simulink model "parkingNavigationTest"  (R2021b)
settings: Solver=VariableStepAuto  StartTime=0.0  StopTime=3600  FixedStep=0.01  RelTol=1e-3
model workspace (MAT data in the model file):
  enableTransmit = 1
libraries: matrix_library x10, sharedutil x4, simulink x3, aerolibutil x2
(part 1 of 2)
settings Model: Creator=Vladik  LastModifiedBy=Vladik

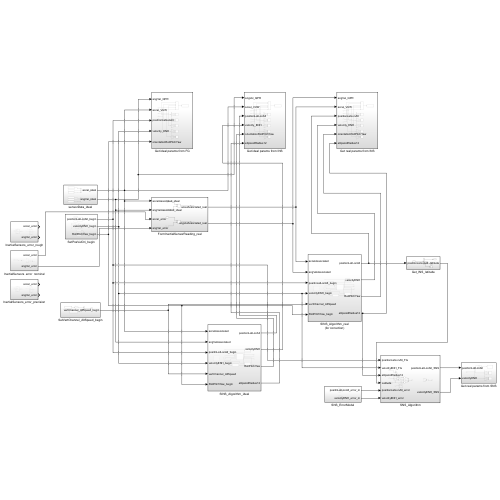
[thumbnail: Simulink's stored preview of the top-level diagram]
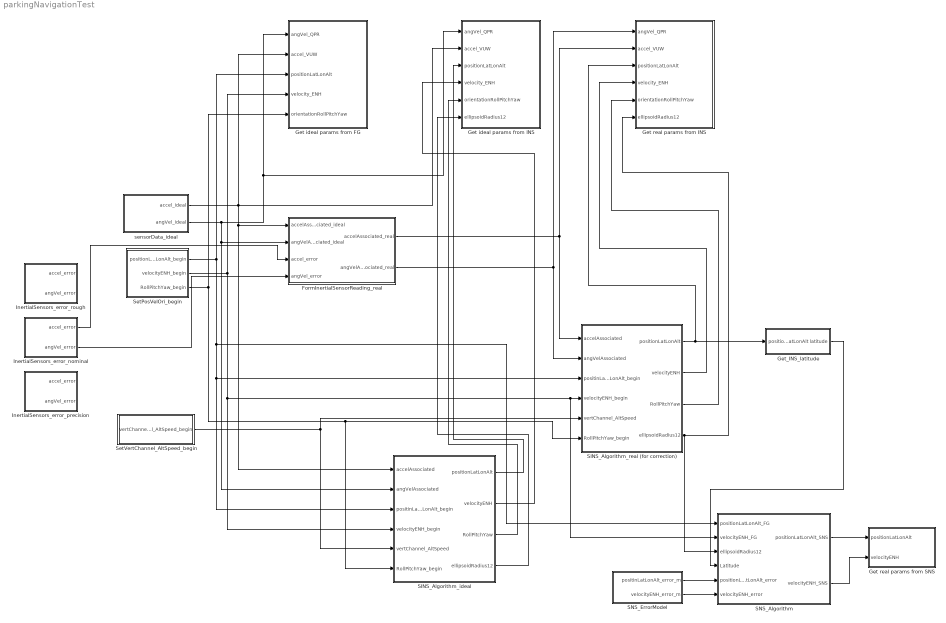
== system parkingNavigationTest ==
  FormInertialSensorReading_real : Subsystem
  Get ideal params from FG : Subsystem
  Get ideal params from INS : Subsystem
  Get real params from INS : Subsystem
  Get real params from SNS : Subsystem
  Get_INS_latitude : Subsystem
  InertialSensors_error_nominal : Subsystem
  InertialSensors_error_precision : Subsystem
  InertialSensors_error_rough : Subsystem
  SINS_Algorithm_ideal : Subsystem
  SINS_Algorithm_real (for correction) : Subsystem
  SNS_Algorithm : Subsystem
  SNS_ErrorModel : Subsystem
  SetPosVelOri_begin : Subsystem
  SetVertChannel_AltSpeed_begin : Subsystem
  sensorData_ideal : Subsystem
  wires:
  SetPosVelOri_begin/2(velocityENH_begin) -> SNS_Algorithm/2(velocityENH_FG), SINS_Algorithm_real (for correction)/4(velocityENH_begin), SINS_Algorithm_ideal/4(velocityENH_begin), Get ideal params from FG/4(velocity_ENH)
  InertialSensors_error_nominal/1(accel_error) -> FormInertialSensorReading_real/3(accel_error)
  InertialSensors_error_nominal/2(angVel_error) -> FormInertialSensorReading_real/4(angVel_error)
  FormInertialSensorReading_real/1(accelAssociated_real) -> SINS_Algorithm_real (for correction)/1(accelAssociated), Get real params from INS/2(accel_VUW)
  FormInertialSensorReading_real/2(angVelAssociated_real) -> SINS_Algorithm_real (for correction)/2(angVelAssociated), Get real params from INS/1(angVel_QPR)
  SetPosVelOri_begin/3(RollPitchYaw_begin) -> SINS_Algorithm_ideal/6(RollPitchYaw_begin), SINS_Algorithm_real (for correction)/6(RollPitchYaw_begin), Get ideal params from FG/5(orientationRollPitchYaw)
  SetPosVelOri_begin/1(positionLatLonAlt_begin) -> SINS_Algorithm_ideal/3(positinLatLonAlt_begin), SINS_Algorithm_real (for correction)/3(positinLatLonAlt_begin), SNS_Algorithm/1(positionLatLonAlt_FG), Get ideal params from FG/3(positionLatLonAlt)
  sensorData_ideal/1(accel_ideal) -> SINS_Algorithm_ideal/1(accelAssociated), FormInertialSensorReading_real/1(accelAssociated_ideal), Get ideal params from FG/2(accel_VUW), Get ideal params from INS/2(accel_VUW)
  SINS_Algorithm_ideal/1(positionLatLonAlt) -> Get ideal params from INS/3(positionLatLonAlt)
  SINS_Algorithm_ideal/2(velocityENH) -> Get ideal params from INS/4(velocity_ENH)
  SINS_Algorithm_ideal/3(RollPitchYaw) -> Get ideal params from INS/5(orientationRollPitchYaw)
  SINS_Algorithm_real (for correction)/1(positionLatLonAlt) -> Get_INS_latitude/1(positionLatLonAlt), Get real params from INS/3(positionLatLonAlt)
  SINS_Algorithm_real (for correction)/3(RollPitchYaw) -> Get real params from INS/5(orientationRollPitchYaw)
  SetVertChannel_AltSpeed_begin/1(vertChannel_AltSpeed_begin) -> SINS_Algorithm_ideal/5(vertChannel_AltSpeed), SINS_Algorithm_real (for correction)/5(vertChannel_AltSpeed)
  SINS_Algorithm_real (for correction)/2(velocityENH) -> Get real params from INS/4(velocity_ENH)
  sensorData_ideal/2(angVel_ideal) -> SINS_Algorithm_ideal/2(angVelAssociated), FormInertialSensorReading_real/2(angVelAssociated_ideal), Get ideal params from INS/1(angVel_QPR), Get ideal params from FG/1(angVel_QPR)
  SINS_Algorithm_ideal/4(ellipsoidRadius12) -> Get ideal params from INS/6(ellipsoidRadius12)
  SINS_Algorithm_real (for correction)/4(ellipsoidRadius12) -> SNS_Algorithm/3(ellipsoidRadius12), Get real params from INS/6(ellipsoidRadius12)
  SNS_ErrorModel/1(positinLatLonAlt_error_m) -> SNS_Algorithm/5(positionLatLonAlt_error)
  SNS_ErrorModel/2(velocityENH_error_m) -> SNS_Algorithm/6(velocityENH_error)
  Get_INS_latitude/1(latitude) -> SNS_Algorithm/4(Latitude)
  SNS_Algorithm/1(positionLatLonAlt_SNS) -> Get real params from SNS/1(positionLatLonAlt)
  SNS_Algorithm/2(velocityENH_SNS) -> Get real params from SNS/2(velocityENH)

== system parkingNavigationTest/FormInertialSensorReading_real ==
  accelAssociated_ideal : Inport
  angVelAssociated_ideal : Inport  Port=2
  accel_error : Inport  Port=3
  angVel_error : Inport  Port=4
  Add : Sum
  Add1 : Sum
  accelAssociated_real : Outport
  angVelAssociated_real : Outport  Port=2
  wires:
  accelAssociated_ideal/1 -> Add/1
  accel_error/1 -> Add/2
  Add/1 -> accelAssociated_real/1
  Add1/1 -> angVelAssociated_real/1
  angVelAssociated_ideal/1 -> Add1/1
  angVel_error/1 -> Add1/2

== system parkingNavigationTest/Get ideal params from FG ==
  angVel_QPR : Inport
  accel_VUW : Inport  Port=2
  positionLatLonAlt : Inport  Port=3
  velocity_ENH : Inport  Port=4
  orientationRollPitchYaw : Inport  Port=5
  Demux{1..5} (5 alike) : Demux  Outputs=3
  Vector Concatenate2 : Concatenate  NumInputs=5  Mode=Multidimensional array
  Write Ideal To File : ToFile  Filename=x_ideal_fg.mat  MatrixName=x_ideal_fg
  dispAccelerationIdeal : Scope  NumInputPorts=3
  dispAngularVelocityIdeal : Scope  NumInputPorts=3
  dispOrientationIdeal : Scope  NumInputPorts=3
  dispPositionIdeal : Scope  NumInputPorts=3
  dispVelocityIdeal : Scope  NumInputPorts=3
  wires:
  Demux3/1 -> dispPositionIdeal/1
  Demux3/3 -> dispPositionIdeal/3
  Demux3/2 -> dispPositionIdeal/2
  positionLatLonAlt/1 -> Demux3/1, Vector Concatenate2/3
  Demux4/1 -> dispVelocityIdeal/1
  Demux4/3 -> dispVelocityIdeal/3
  Demux4/2 -> dispVelocityIdeal/2
  velocity_ENH/1 -> Vector Concatenate2/4, Demux4/1
  Demux5/1 -> dispOrientationIdeal/1
  Demux5/2 -> dispOrientationIdeal/2
  Demux5/3 -> dispOrientationIdeal/3
  orientationRollPitchYaw/1 -> Vector Concatenate2/5, Demux5/1
  Demux1/3 -> dispAccelerationIdeal/3
  Demux1/1 -> dispAccelerationIdeal/1
  Demux1/2 -> dispAccelerationIdeal/2
  accel_VUW/1 -> Demux1/1, Vector Concatenate2/2
  Demux2/3 -> dispAngularVelocityIdeal/3
  Demux2/1 -> dispAngularVelocityIdeal/1
  Demux2/2 -> dispAngularVelocityIdeal/2
  angVel_QPR/1 -> Vector Concatenate2/1, Demux2/1
  Vector Concatenate2/1 -> Write Ideal To File/1

== system parkingNavigationTest/Get ideal params from INS ==
  angVel_QPR : Inport
  accel_VUW : Inport  Port=2
  positionLatLonAlt : Inport  Port=3
  velocity_ENH : Inport  Port=4
  orientationRollPitchYaw : Inport  Port=5
  ellipsoidRadius12 : Inport  Port=6
  Demux{1..5} (5 alike) : Demux  Outputs=3
  Vector Concatenate2 : Concatenate  NumInputs=6  Mode=Multidimensional array
  Write Ideal To File : ToFile  Filename=x_ideal_ins.mat  MatrixName=x_ideal_ins
  dispAccelerationIdeal_INS : Scope  NumInputPorts=3
  dispAngularVelocityIdeal_INS : Scope  NumInputPorts=3
  dispOrientationIdeal_INS : Scope  NumInputPorts=3
  dispPositionIdeal_INS : Scope  NumInputPorts=3
  dispVelocityIdeal_INS : Scope  NumInputPorts=3
  wires:
  Demux3/1 -> dispPositionIdeal_INS/1
  Demux3/3 -> dispPositionIdeal_INS/3
  Demux3/2 -> dispPositionIdeal_INS/2
  positionLatLonAlt/1 -> Vector Concatenate2/3, Demux3/1
  Demux4/1 -> dispVelocityIdeal_INS/1
  Demux4/3 -> dispVelocityIdeal_INS/3
  Demux4/2 -> dispVelocityIdeal_INS/2
  velocity_ENH/1 -> Vector Concatenate2/4, Demux4/1
  Demux5/1 -> dispOrientationIdeal_INS/1
  Demux5/2 -> dispOrientationIdeal_INS/2
  Demux5/3 -> dispOrientationIdeal_INS/3
  orientationRollPitchYaw/1 -> Vector Concatenate2/5, Demux5/1
  Demux1/3 -> dispAccelerationIdeal_INS/3
  Demux1/1 -> dispAccelerationIdeal_INS/1
  Demux1/2 -> dispAccelerationIdeal_INS/2
  accel_VUW/1 -> Vector Concatenate2/2, Demux1/1
  Demux2/3 -> dispAngularVelocityIdeal_INS/3
  Demux2/1 -> dispAngularVelocityIdeal_INS/1
  Demux2/2 -> dispAngularVelocityIdeal_INS/2
  angVel_QPR/1 -> Vector Concatenate2/1, Demux2/1
  Vector Concatenate2/1 -> Write Ideal To File/1
  ellipsoidRadius12/1 -> Vector Concatenate2/6

== system parkingNavigationTest/Get real params from INS ==
  angVel_QPR : Inport
  accel_VUW : Inport  Port=2
  positionLatLonAlt : Inport  Port=3
  velocity_ENH : Inport  Port=4
  orientationRollPitchYaw : Inport  Port=5
  ellipsoidRadius12 : Inport  Port=6
  Demux{1..5} (5 alike) : Demux  Outputs=3
  Vector Concatenate2 : Concatenate  NumInputs=6  Mode=Multidimensional array
  Write Real To File : ToFile  Filename=x_real_ins.mat  MatrixName=x_real_ins
  dispAccelerationReal_INS : Scope  NumInputPorts=3
  dispAngularVelocityReal_INS : Scope  NumInputPorts=3
  dispOrientationReal_INS : Scope  NumInputPorts=3
  dispPositionReal_INS : Scope  NumInputPorts=3
  dispVelocityReal_INS : Scope  NumInputPorts=3
  wires:
  Demux3/1 -> dispPositionReal_INS/1
  Demux3/3 -> dispPositionReal_INS/3
  Demux3/2 -> dispPositionReal_INS/2
  positionLatLonAlt/1 -> Vector Concatenate2/3, Demux3/1
  Demux4/1 -> dispVelocityReal_INS/1
  Demux4/3 -> dispVelocityReal_INS/3
  Demux4/2 -> dispVelocityReal_INS/2
  velocity_ENH/1 -> Vector Concatenate2/4, Demux4/1
  Demux5/1 -> dispOrientationReal_INS/1
  Demux5/2 -> dispOrientationReal_INS/2
  Demux5/3 -> dispOrientationReal_INS/3
  orientationRollPitchYaw/1 -> Vector Concatenate2/5, Demux5/1
  Demux1/3 -> dispAccelerationReal_INS/3
  Demux1/1 -> dispAccelerationReal_INS/1
  Demux1/2 -> dispAccelerationReal_INS/2
  accel_VUW/1 -> Vector Concatenate2/2, Demux1/1
  Demux2/3 -> dispAngularVelocityReal_INS/3
  Demux2/1 -> dispAngularVelocityReal_INS/1
  Demux2/2 -> dispAngularVelocityReal_INS/2
  angVel_QPR/1 -> Vector Concatenate2/1, Demux2/1
  Vector Concatenate2/1 -> Write Real To File/1
  ellipsoidRadius12/1 -> Vector Concatenate2/6

== system parkingNavigationTest/Get real params from SNS ==
  positionLatLonAlt : Inport
  velocityENH : Inport  Port=2
  Demux3 : Demux  Outputs=3
  Demux4 : Demux  Outputs=3
  Vector Concatenate2 : Concatenate  Mode=Multidimensional array
  Write Data To File : ToFile  Filename=x_real_sns.mat  MatrixName=x_real_sns
  dispPosition : Scope  NumInputPorts=3
  dispVelocity : Scope  NumInputPorts=3
  wires:
  positionLatLonAlt/1 -> Vector Concatenate2/1, Demux3/1
  Vector Concatenate2/1 -> Write Data To File/1
  Demux3/2 -> dispPosition/2
  Demux3/3 -> dispPosition/3
  Demux3/1 -> dispPosition/1
  velocityENH/1 -> Vector Concatenate2/2, Demux4/1
  Demux4/1 -> dispVelocity/1
  Demux4/2 -> dispVelocity/2
  Demux4/3 -> dispVelocity/3

== system parkingNavigationTest/Get_INS_latitude ==
  positionLatLonAlt : Inport
  Demux : Demux  Outputs=3
  Terminator : Terminator
  Terminator1 : Terminator
  latitude : Outport
  wires:
  positionLatLonAlt/1 -> Demux/1
  Demux/1 -> latitude/1
  Demux/2 -> Terminator/1
  Demux/3 -> Terminator1/1

== system parkingNavigationTest/InertialSensors_error_nominal ==
  Add1 : Sum
  Add4 : Sum
  Mux : Mux  Inputs=3
  Mux1 : Mux  Inputs=3
  Ramp : simulink/Sources/Ramp  slope=0.015*pi/180/3600  start=0  InitialOutput=0
  accelNoise : RandomNumber  Variance=1e-8  SampleTime=1
  accelZeroOffset : Constant  Value=5e-4
  gyroNoise : RandomNumber  Variance=(0.01*pi/180/3600)^2  SampleTime=1
  accel_error : Outport
  angVel_error : Outport  Port=2
  wires:
  gyroNoise/1 -> Add4/2
  accelZeroOffset/1 -> Add1/1
  accelNoise/1 -> Add1/2
  Add1/1 -> Mux/1, Mux/2, Mux/3
  Mux/1 -> accel_error/1
  Mux1/1 -> angVel_error/1
  Ramp/1 -> Add4/1
  Add4/1 -> Mux1/1, Mux1/2, Mux1/3

== system parkingNavigationTest/InertialSensors_error_precision ==
  Add{,1..5} (6 alike) : Sum
  Mux : Mux  Inputs=3
  Mux1 : Mux  Inputs=3
  Ramp : simulink/Sources/Ramp  slope=0.0015*pi/180/3600  start=0  InitialOutput=0
  accelNoise : RandomNumber  Variance=1e-10  SampleTime=1
  accelZeroOffset : Constant  Value=0.00005
  gyroNoise : RandomNumber  Variance=(0.001*pi/180/3600)^2  SampleTime=1
  accel_error : Outport
  angVel_error : Outport  Port=2
  wires:
  gyroNoise/1 -> Add/2, Add5/2, Add4/2
  accelZeroOffset/1 -> Add2/1, Add3/1, Add1/1
  accelNoise/1 -> Add3/2, Add2/2, Add1/2
  Add1/1 -> Mux/2
  Mux/1 -> accel_error/1
  Mux1/1 -> angVel_error/1
  Add2/1 -> Mux/1
  Add3/1 -> Mux/3
  Ramp/1 -> Add5/1, Add4/1, Add/1
  Add4/1 -> Mux1/2
  Add/1 -> Mux1/1
  Add5/1 -> Mux1/3

== system parkingNavigationTest/InertialSensors_error_rough ==
  Add{,1..5} (6 alike) : Sum
  Mux : Mux  Inputs=3
  Mux1 : Mux  Inputs=3
  Ramp : simulink/Sources/Ramp  slope=0.15*pi/180/3600  start=0  InitialOutput=0
  accelNoise : RandomNumber  Variance=1e-6  SampleTime=1
  accelZeroOffset : Constant  Value=5e-3
  gyroNoise : RandomNumber  Variance=(0.1*pi/180/3600)^2  SampleTime=1
  accel_error : Outport
  angVel_error : Outport  Port=2
  wires:
  gyroNoise/1 -> Add/2, Add5/2, Add4/2
  accelZeroOffset/1 -> Add2/1, Add3/1, Add1/1
  accelNoise/1 -> Add3/2, Add2/2, Add1/2
  Add1/1 -> Mux/2
  Mux/1 -> accel_error/1
  Mux1/1 -> angVel_error/1
  Add2/1 -> Mux/1
  Add3/1 -> Mux/3
  Ramp/1 -> Add5/1, Add4/1, Add/1
  Add4/1 -> Mux1/2
  Add/1 -> Mux1/1
  Add5/1 -> Mux1/3

== system parkingNavigationTest/SINS_Algorithm_ideal ==
  accelAssociated : Inport
  angVelAssociated : Inport  Port=2
  positinLatLonAlt_begin : Inport  Port=3
  velocityENH_begin : Inport  Port=4
  vertChannel_AltSpeed : Inport  Port=5
  RollPitchYaw_begin : Inport  Port=6
  CalculateAccelerationsXYZ : Subsystem
  GetC_begin_easy : Subsystem
  GetC_begin_vectorMatching : Subsystem  Commented=on
  NavigationAlgorithm : Subsystem
  OrientationAlgorithm : Subsystem
  U_earth : Constant  Value=7.29212e-5
  removeVelocityH : Subsystem
  positionLatLonAlt : Outport
  velocityENH : Outport  Port=2
  RollPitchYaw : Outport  Port=3
  ellipsoidRadius12 : Outport  Port=4
  wires:
  GetC_begin_easy/1(C_assoc_norm_begin) -> OrientationAlgorithm/3(C_assoc_norm_begin)
  velocityENH_begin/1 -> removeVelocityH/1(velocityENH_begin)
  NavigationAlgorithm/4(ellipsoidRadius12) -> ellipsoidRadius12/1
  vertChannel_AltSpeed/1 -> NavigationAlgorithm/5(vertChannel_AltSpeed)
  NavigationAlgorithm/2(velocityENH) -> velocityENH/1
  removeVelocityH/1(velocityEN_begin) -> NavigationAlgorithm/3(velocityEN_begin)
  positinLatLonAlt_begin/1 -> NavigationAlgorithm/2(positionLatLonAlt_begin)
  NavigationAlgorithm/3(angVelNorm_matrix_3x3) -> OrientationAlgorithm/2(angVelNorm_matrix)
  NavigationAlgorithm/1(positionLatLonAlt) -> positionLatLonAlt/1
  U_earth/1 -> NavigationAlgorithm/4(U_earth)
  angVelAssociated/1 -> OrientationAlgorithm/1(angVel_inertial_assoc)
  OrientationAlgorithm/1(C_assoc_norm) -> CalculateAccelerationsXYZ/2(C_accoc_norm)
  accelAssociated/1 -> CalculateAccelerationsXYZ/1(accelerationAssociated)
  RollPitchYaw_begin/1 -> GetC_begin_easy/1(RollPitchYaw_begin)
  OrientationAlgorithm/2(RollPitchYaw) -> RollPitchYaw/1
  CalculateAccelerationsXYZ/1(accelerationXYZ) -> NavigationAlgorithm/1(accelerationXYZ)

== system parkingNavigationTest/SINS_Algorithm_real (for correction) ==
  accelAssociated : Inport
  angVelAssociated : Inport  Port=2
  positinLatLonAlt_begin : Inport  Port=3
  velocityENH_begin : Inport  Port=4
  vertChannel_AltSpeed : Inport  Port=5
  RollPitchYaw_begin : Inport  Port=6
  CalculateAccelerationsXYZ : Subsystem
  GetC_begin_easy : Subsystem
  GetC_begin_vectorMatching : Subsystem  Commented=on
  NavigationAlgorithm : Subsystem
  OrientationAlgorithm : Subsystem
  U_earth : Constant  Value=7.29212e-5
  removeVelocityH : Subsystem
  positionLatLonAlt : Outport
  velocityENH : Outport  Port=2
  RollPitchYaw : Outport  Port=3
  ellipsoidRadius12 : Outport  Port=4
  wires:
  NavigationAlgorithm/2(velocityENH) -> velocityENH/1
  CalculateAccelerationsXYZ/1(accelerationXYZ) -> NavigationAlgorithm/1(accelerationXYZ)
  positinLatLonAlt_begin/1 -> NavigationAlgorithm/2(positionLatLonAlt_begin)
  removeVelocityH/1(velocityEN_begin) -> NavigationAlgorithm/3(velocityEN_begin)
  velocityENH_begin/1 -> removeVelocityH/1(velocityENH_begin)
  GetC_begin_easy/1(C_assoc_norm_begin) -> OrientationAlgorithm/3(C_assoc_norm_begin)
  vertChannel_AltSpeed/1 -> NavigationAlgorithm/5(vertChannel_AltSpeed)
  U_earth/1 -> NavigationAlgorithm/4(U_earth)
  NavigationAlgorithm/4(ellipsoidRadius12) -> ellipsoidRadius12/1
  OrientationAlgorithm/1(C_assoc_norm) -> CalculateAccelerationsXYZ/2(C_accoc_norm)
  accelAssociated/1 -> CalculateAccelerationsXYZ/1(accelerationAssociated)
  NavigationAlgorithm/3(angVelNorm_matrix_3x3) -> OrientationAlgorithm/2(angVelNorm_matrix)
  OrientationAlgorithm/2(RollPitchYaw) -> RollPitchYaw/1
  NavigationAlgorithm/1(positionLatLonAlt) -> positionLatLonAlt/1
  angVelAssociated/1 -> OrientationAlgorithm/1(angVel_inertial_assoc)
  RollPitchYaw_begin/1 -> GetC_begin_easy/1(RollPitchYaw_begin)

== system parkingNavigationTest/SNS_Algorithm ==
  positionLatLonAlt_FG : Inport
  velocityENH_FG : Inport  Port=2
  ellipsoidRadius12 : Inport  Port=3
  Latitude : Inport  Port=4
  positionLatLonAlt_error : Inport  Port=5
  velocityENH_error : Inport  Port=6
  Add1 : Sum
  AltReal_m : Sum
  Cos : Trigonometry  Operator=cos
  Demux1 : Demux  Outputs=3
  Demux7 : Demux  Outputs=3
  Demux8 : Demux  Outputs=2
  Divide : Product  Inputs=*/
  Divide1 : Product  Inputs=*//
  LatSNS_rad : Sum
  LonReal_rad : Sum
  Mux2 : Mux  Inputs=3
  positionLatLonAlt_SNS : Outport
  velocityENH_SNS : Outport  Port=2
  wires:
  Divide1/1 -> LonReal_rad/1
  Divide/1 -> LatSNS_rad/1
  ellipsoidRadius12/1 -> Demux8/1
  positionLatLonAlt_error/1 -> Demux7/1
  Demux7/1 -> Divide/1
  Demux7/2 -> Divide1/1
  Latitude/1 -> Cos/1
  Cos/1 -> Divide1/3
  positionLatLonAlt_FG/1 -> Demux1/1
  Demux1/1 -> LatSNS_rad/2
  Demux1/2 -> LonReal_rad/2
  Demux7/3 -> AltReal_m/1
  Demux1/3 -> AltReal_m/2
  LonReal_rad/1 -> Mux2/2
  LatSNS_rad/1 -> Mux2/1
  AltReal_m/1 -> Mux2/3
  Mux2/1 -> positionLatLonAlt_SNS/1
  velocityENH_FG/1 -> Add1/1
  velocityENH_error/1 -> Add1/2
  Add1/1 -> velocityENH_SNS/1
  Demux8/2 -> Divide/2
  Demux8/1 -> Divide1/2

== system parkingNavigationTest/SNS_ErrorModel ==
  AltError_m : RandomNumber  Variance=100  SampleTime=0.1
  LatError_m : RandomNumber  Variance=100  SampleTime=0.1
  LonError_m : RandomNumber  Variance=100  SampleTime=0.1
  Mux : Mux  Inputs=3
  Mux1 : Mux  Inputs=3
  VelE_error_m : RandomNumber  Variance=0.01  SampleTime=0.1
  VelH_error_m : RandomNumber  Variance=0.01  SampleTime=0.1
  VelN_error_m : RandomNumber  Variance=0.01  SampleTime=0.1
  positinLatLonAlt_error_m : Outport
  velocityENH_error_m : Outport  Port=2
  wires:
  LonError_m/1 -> Mux/2
  LatError_m/1 -> Mux/1
  AltError_m/1 -> Mux/3
  Mux/1 -> positinLatLonAlt_error_m/1
  VelN_error_m/1 -> Mux1/2
  VelE_error_m/1 -> Mux1/1
  VelH_error_m/1 -> Mux1/3
  Mux1/1 -> velocityENH_error_m/1

== system parkingNavigationTest/SetPosVelOri_begin ==
  Gain : Gain  Gain=0.3048
  Gain1 : Gain  Gain=0.3048
  Gain2 : Gain  Gain=0.3048
  Mux : Mux  Inputs=3
  Mux1 : Mux  Inputs=3
  Mux2 : Mux  Inputs=3
  Pitch_begin : Constant  Value=0
  Roll_begin : Constant  Value=0
  Yaw_begin : Constant  Value=0
  altitude_ft_begin : Constant  Value=177.0373066799141
  latitude_deg_begin : Constant  Value=0.9672608180643483
  longitude_deg_begin : Constant  Value=0.6611314818805803
  velocityE_mps_begin : Constant  Value=0
  velocityH_mps_begin : Constant  Value=0
  velocityN_mps_begin : Constant  Value=0
  positionLatLonAlt_begin : Outport
  velocityENH_begin : Outport  Port=2
  RollPitchYaw_begin : Outport  Port=3
  wires:
  Mux1/1 -> velocityENH_begin/1
  longitude_deg_begin/1 -> Mux/2
  altitude_ft_begin/1 -> Mux/3
  latitude_deg_begin/1 -> Mux/1
  Mux/1 -> positionLatLonAlt_begin/1
  Yaw_begin/1 -> Mux2/3
  Pitch_begin/1 -> Mux2/2
  Roll_begin/1 -> Mux2/1
  Mux2/1 -> RollPitchYaw_begin/1
  Gain/1 -> Mux1/1
  velocityE_mps_begin/1 -> Gain/1
  velocityN_mps_begin/1 -> Gain1/1
  Gain1/1 -> Mux1/2
  velocityH_mps_begin/1 -> Gain2/1
  Gain2/1 -> Mux1/3

== system parkingNavigationTest/SetVertChannel_AltSpeed_begin ==
  Mux : Mux  Inputs=2
  altitude_ft_begin : Constant  Value=518.4845702909249
  feet to meters : Gain  Gain=0.3048
  velocityH_mps_begin : Constant  Value=0.06847562969267891
  vertChannel_AltSpeed_begin : Outport
  wires:
  velocityH_mps_begin/1 -> Mux/2
  feet to meters/1 -> Mux/1
  altitude_ft_begin/1 -> feet to meters/1
  Mux/1 -> vertChannel_AltSpeed_begin/1

== system parkingNavigationTest/sensorData_ideal ==
  Constant{,1..5} (6 alike) : Constant  Value=0
  Mux : Mux  Inputs=3
  Mux1 : Mux  Inputs=3
  accel_ideal : Outport
  angVel_ideal : Outport  Port=2
  wires:
  Constant2/1 -> Mux/1
  Constant/1 -> Mux/2
  Constant1/1 -> Mux/3
  Constant5/1 -> Mux1/1
  Constant3/1 -> Mux1/2
  Constant4/1 -> Mux1/3
  Mux1/1 -> angVel_ideal/1
  Mux/1 -> accel_ideal/1

== system parkingNavigationTest/SINS_Algorithm_ideal/CalculateAccelerationsXYZ ==
  accelerationAssociated : Inport
  C_accoc_norm : Inport  Port=2
  Product : Product  Multiplication=Matrix(*)
  accelerationXYZ : Outport
  wires:
  accelerationAssociated/1 -> Product/2
  Product/1 -> accelerationXYZ/1
  C_accoc_norm/1 -> Product/1

== system parkingNavigationTest/SINS_Algorithm_ideal/GetC_begin_easy ==
  RollPitchYaw_begin : Inport
  Cos2 : Trigonometry  Operator=cos
  Mux1 : Mux  Inputs=2
  Sin2 : Trigonometry
  calculate C_begin : MATLAB Function  TreatAsAtomicUnit=on
  C_assoc_norm_begin : Outport
  wires:
  RollPitchYaw_begin/1 -> Sin2/1, Cos2/1
  Sin2/1 -> Mux1/1
  Cos2/1 -> Mux1/2
  Mux1/1 -> calculate C_begin/1(u)
  calculate C_begin/1(y) -> C_assoc_norm_begin/1

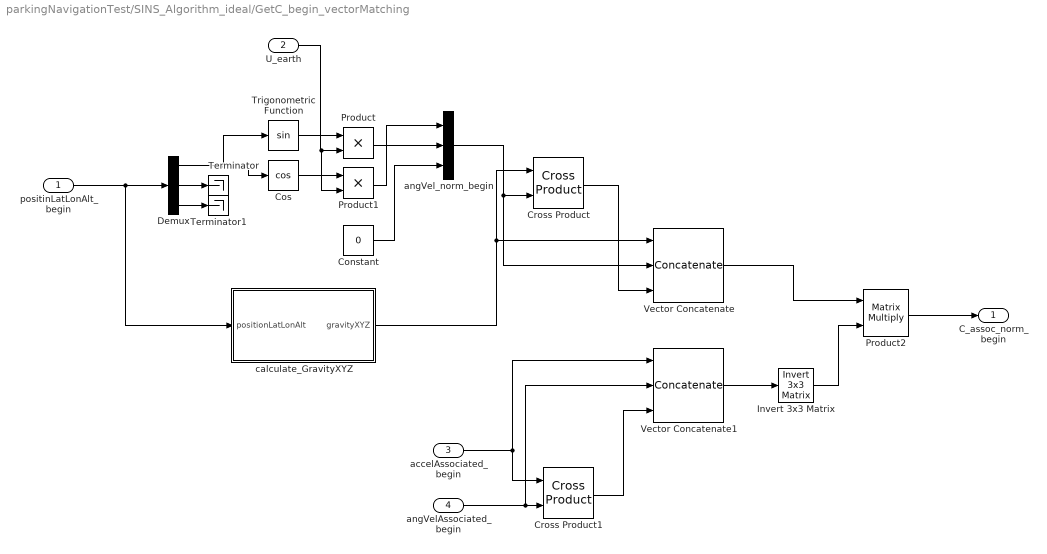
== system parkingNavigationTest/SINS_Algorithm_ideal/GetC_begin_vectorMatching ==
  positinLatLonAlt_begin : Inport
  U_earth : Inport  Port=2
  accelAssociated_begin : Inport  Port=3
  angVelAssociated_begin : Inport  Port=4
  Constant : Constant  Value=0
  Cos : Trigonometry  Operator=cos
  Cross Product : matrix_library/Cross Product
      settings: SourceProductBaseCode=SL
  Cross Product1 : matrix_library/Cross Product
      settings: SourceProductBaseCode=SL
  Demux : Demux  Outputs=3
  Invert 3x3 Matrix : aerolibutil/Invert  3x3 Matrix
  Product : Product
  Product1 : Product
  Product2 : Product  Multiplication=Matrix(*)
  Terminator : Terminator
  Terminator1 : Terminator
  Trigonometric Function : Trigonometry
  Vector Concatenate : Concatenate  NumInputs=3  Mode=Multidimensional array  ConcatenateDimension=2
  Vector Concatenate1 : Concatenate  NumInputs=3  Mode=Multidimensional array  ConcatenateDimension=2
  angVel_norm_begin : Mux  Inputs=3
  calculate_GravityXYZ : Subsystem
  C_assoc_norm_begin : Outport
  wires:
  Trigonometric Function/1 -> Product/1
  Demux/1 -> Cos/1, Trigonometric Function/1
  Cos/1 -> Product1/1
  Constant/1 -> angVel_norm_begin/3
  Product/1 -> angVel_norm_begin/2
  Product1/1 -> angVel_norm_begin/1
  Demux/3 -> Terminator1/1
  Demux/2 -> Terminator/1
  calculate_GravityXYZ/1(gravityXYZ) -> Vector Concatenate/1, Cross Product/1
  angVel_norm_begin/1 -> Vector Concatenate/2, Cross Product/2
  positinLatLonAlt_begin/1 -> calculate_GravityXYZ/1(positionLatLonAlt), Demux/1
  U_earth/1 -> Product1/2, Product/2
  Cross Product/1 -> Vector Concatenate/3
  accelAssociated_begin/1 -> Vector Concatenate1/1, Cross Product1/1
  angVelAssociated_begin/1 -> Vector Concatenate1/2, Cross Product1/2
  Cross Product1/1 -> Vector Concatenate1/3
  Vector Concatenate1/1 -> Invert 3x3 Matrix/1
  Vector Concatenate/1 -> Product2/1
  Invert 3x3 Matrix/1 -> Product2/2
  Product2/1 -> C_assoc_norm_begin/1

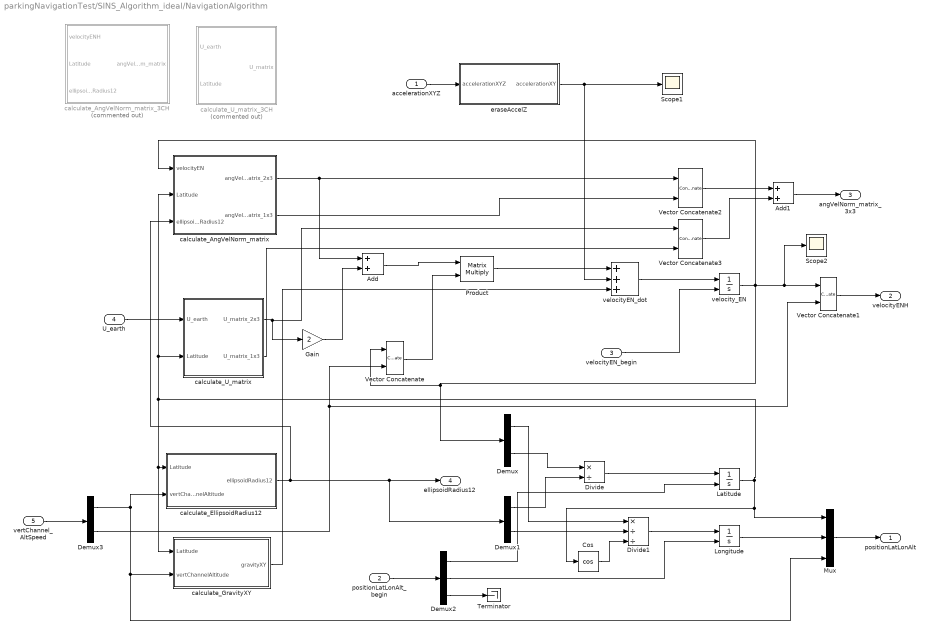
== system parkingNavigationTest/SINS_Algorithm_ideal/NavigationAlgorithm ==
  accelerationXYZ : Inport
  positionLatLonAlt_begin : Inport  Port=2
  velocityEN_begin : Inport  Port=3
  U_earth : Inport  Port=4
  vertChannel_AltSpeed : Inport  Port=5
  Add : Sum
  Add1 : Sum
  Cos : Trigonometry  Operator=cos
  Demux : Demux  Outputs=2
  Demux1 : Demux  Outputs=2
  Demux2 : Demux  Outputs=3
  Demux3 : Demux  Outputs=2
  Divide : Product  Inputs=*/
  Divide1 : Product  Inputs=*//
  Gain : Gain  Gain=2
  Latitude : Integrator  InitialConditionSource=external
  Longitude : Integrator  InitialConditionSource=external
  Mux : Mux  Inputs=3
  Product : Product  Multiplication=Matrix(*)
  Scope1 : Scope
  Scope2 : Scope
  Terminator : Terminator
  Vector Concatenate{,1..3} (4 alike) : Concatenate  Mode=Multidimensional array
  calculate_AngVelNorm_matrix : Subsystem
  calculate_AngVelNorm_matrix_3CH : Subsystem  Commented=on
  calculate_EllipsoidRadius12 : Subsystem
  calculate_GravityXY : Subsystem
  calculate_U_matrix : Subsystem
  calculate_U_matrix_3CH : Subsystem  Commented=on
  eraseAccelZ : Subsystem
  velocityEN_dot : Sum  Inputs=+++
  velocity_EN : Integrator  InitialConditionSource=external  InitialCondition=[0; 0; 0]
  positionLatLonAlt : Outport
  velocityENH : Outport  Port=2
  angVelNorm_matrix_3x3 : Outport  Port=3
  ellipsoidRadius12 : Outport  Port=4
  wires:
  calculate_U_matrix/1(U_matrix_2x3) -> Vector Concatenate3/1, Gain/1
  calculate_AngVelNorm_matrix/1(angVelNorm_matrix_2x3) -> Vector Concatenate2/1, Add/1
  Gain/1 -> Add/2
  Add/1 -> Product/1
  Product/1 -> velocityEN_dot/1
  velocityEN_dot/1 -> velocity_EN/1
  Divide/1 -> Latitude/1
  Demux/2 -> Divide/1
  Demux1/1 -> Divide/2
  Latitude/1 -> calculate_GravityXY/1(Latitude), calculate_EllipsoidRadius12/1(Latitude), calculate_U_matrix/2(Latitude), calculate_AngVelNorm_matrix/2(Latitude), Mux/1, Cos/1
  Divide1/1 -> Longitude/1
  Demux/1 -> Divide1/1
  Demux1/2 -> Divide1/2
  Cos/1 -> Divide1/3
  Longitude/1 -> Mux/2
  Demux3/1 -> Mux/3, calculate_GravityXY/2(vertChannelAltitude), calculate_EllipsoidRadius12/2(vertChannelAltitude)
  calculate_EllipsoidRadius12/1(ellipsoidRadius12) -> calculate_AngVelNorm_matrix/3(ellipsoidRadius12), ellipsoidRadius12/1, Demux1/1
  U_earth/1 -> calculate_U_matrix/1(U_earth)
  Mux/1 -> positionLatLonAlt/1
  velocity_EN/1 -> Scope2/1, Vector Concatenate1/1, calculate_AngVelNorm_matrix/1(velocityEN), Vector Concatenate/1, Demux/1
  calculate_GravityXY/1(gravityXY) -> velocityEN_dot/3
  positionLatLonAlt_begin/1 -> Demux2/1
  Demux2/1 -> Latitude/2
  Demux2/2 -> Longitude/2
  velocityEN_begin/1 -> velocity_EN/2
  vertChannel_AltSpeed/1 -> Demux3/1
  Demux3/2 -> Vector Concatenate1/2, Vector Concatenate/2
  Vector Concatenate/1 -> Product/2
  Vector Concatenate1/1 -> velocityENH/1
  calculate_AngVelNorm_matrix/2(angVelNorm_matrix_1x3) -> Vector Concatenate2/2
  accelerationXYZ/1 -> eraseAccelZ/1(accelerationXYZ)
  eraseAccelZ/1(accelerationXY) -> Scope1/1, velocityEN_dot/2
  Demux2/3 -> Terminator/1
  calculate_U_matrix/2(U_matrix_1x3) -> Vector Concatenate3/2
  Vector Concatenate2/1 -> Add1/1
  Vector Concatenate3/1 -> Add1/2
  Add1/1 -> angVelNorm_matrix_3x3/1

== system parkingNavigationTest/SINS_Algorithm_ideal/OrientationAlgorithm ==
  angVel_inertial_assoc : Inport
  angVelNorm_matrix : Inport  Port=2
  C_assoc_norm_begin : Inport  Port=3
  C to Orientation Angles : Subsystem
  Constant2 : Constant  Value=[1 0 0; 0 1 0; 0 0 1]
  Demux : Demux  Outputs=3
  Integrator : Integrator  InitialConditionSource=external  InitialCondition=[0, 0, 0; 0, 0, 0; 0, 0, 0]
  Product : Product  Multiplication=Matrix(*)
  Product1 : Product  Multiplication=Matrix(*)
  "Skew symmetric matrix " : Subsystem
  Sum : Sum  Inputs=+-
  Transpose : matrix_library/Transpose
      settings: SourceProductBaseCode=SL
  C_assoc_norm : Outport
  RollPitchYaw : Outport  Port=2
  wires:
  angVel_inertial_assoc/1 -> Demux/1
  angVelNorm_matrix/1 -> Transpose/1
  Sum/1 -> Integrator/1
  Transpose/1 -> Product1/1
  Product/1 -> Sum/1
  Product1/1 -> Sum/2
  Integrator/1 -> C to Orientation Angles/1(C), Product/1, Product1/2, C_assoc_norm/1
  C to Orientation Angles/1(RollPitchYaw) -> RollPitchYaw/1
  Demux/2 -> "Skew symmetric matrix "/2(angVel_y)
  Demux/1 -> "Skew symmetric matrix "/1(angVel_x)
  Demux/3 -> "Skew symmetric matrix "/3(angVel_z)
  "Skew symmetric matrix "/1(angVel_matrix) -> Product/2
  C_assoc_norm_begin/1 -> Integrator/2

== system parkingNavigationTest/SINS_Algorithm_ideal/removeVelocityH ==
  velocityENH_begin : Inport
  Demux : Demux  Outputs=3
  Mux : Mux  Inputs=2
  Terminator : Terminator
  velocityEN_begin : Outport
  wires:
  velocityENH_begin/1 -> Demux/1
  Demux/1 -> Mux/1
  Demux/2 -> Mux/2
  Mux/1 -> velocityEN_begin/1
  Demux/3 -> Terminator/1

== system parkingNavigationTest/SINS_Algorithm_real (for correction)/CalculateAccelerationsXYZ ==
  accelerationAssociated : Inport
  C_accoc_norm : Inport  Port=2
  Product : Product  Multiplication=Matrix(*)
  accelerationXYZ : Outport
  wires:
  accelerationAssociated/1 -> Product/2
  Product/1 -> accelerationXYZ/1
  C_accoc_norm/1 -> Product/1

== system parkingNavigationTest/SINS_Algorithm_real (for correction)/GetC_begin_easy ==
  RollPitchYaw_begin : Inport
  Cos2 : Trigonometry  Operator=cos
  Mux1 : Mux  Inputs=2
  Sin2 : Trigonometry
  calculate C_begin : MATLAB Function  TreatAsAtomicUnit=on
  C_assoc_norm_begin : Outport
  wires:
  RollPitchYaw_begin/1 -> Sin2/1, Cos2/1
  Sin2/1 -> Mux1/1
  Cos2/1 -> Mux1/2
  Mux1/1 -> calculate C_begin/1(u)
  calculate C_begin/1(y) -> C_assoc_norm_begin/1

== system parkingNavigationTest/SINS_Algorithm_real (for correction)/GetC_begin_vectorMatching ==
  positinLatLonAlt_begin : Inport
  U_earth : Inport  Port=2
  accelAssociated_begin : Inport  Port=3
  angVelAssociated_begin : Inport  Port=4
  Constant : Constant  Value=0
  Cos : Trigonometry  Operator=cos
  Cross Product : matrix_library/Cross Product
      settings: SourceProductBaseCode=SL
  Cross Product1 : matrix_library/Cross Product
      settings: SourceProductBaseCode=SL
  Demux : Demux  Outputs=3
  Invert 3x3 Matrix : aerolibutil/Invert  3x3 Matrix
  Product : Product
  Product1 : Product
  Product2 : Product  Multiplication=Matrix(*)
  Terminator : Terminator
  Terminator1 : Terminator
  Trigonometric Function : Trigonometry
  Vector Concatenate : Concatenate  NumInputs=3  Mode=Multidimensional array  ConcatenateDimension=2
  Vector Concatenate1 : Concatenate  NumInputs=3  Mode=Multidimensional array  ConcatenateDimension=2
  angVel_norm_begin : Mux  Inputs=3
  calculate_GravityXYZ : Subsystem
  C_assoc_norm_begin : Outport
  wires:
  Trigonometric Function/1 -> Product/1
  Demux/1 -> Cos/1, Trigonometric Function/1
  Cos/1 -> Product1/1
  Constant/1 -> angVel_norm_begin/3
  Product/1 -> angVel_norm_begin/2
  Product1/1 -> angVel_norm_begin/1
  Demux/3 -> Terminator1/1
  Demux/2 -> Terminator/1
  calculate_GravityXYZ/1(gravityXYZ) -> Vector Concatenate/1, Cross Product/1
  angVel_norm_begin/1 -> Vector Concatenate/2, Cross Product/2
  positinLatLonAlt_begin/1 -> calculate_GravityXYZ/1(positionLatLonAlt), Demux/1
  U_earth/1 -> Product1/2, Product/2
  Cross Product/1 -> Vector Concatenate/3
  accelAssociated_begin/1 -> Vector Concatenate1/1, Cross Product1/1
  angVelAssociated_begin/1 -> Vector Concatenate1/2, Cross Product1/2
  Cross Product1/1 -> Vector Concatenate1/3
  Vector Concatenate1/1 -> Invert 3x3 Matrix/1
  Vector Concatenate/1 -> Product2/1
  Invert 3x3 Matrix/1 -> Product2/2
  Product2/1 -> C_assoc_norm_begin/1

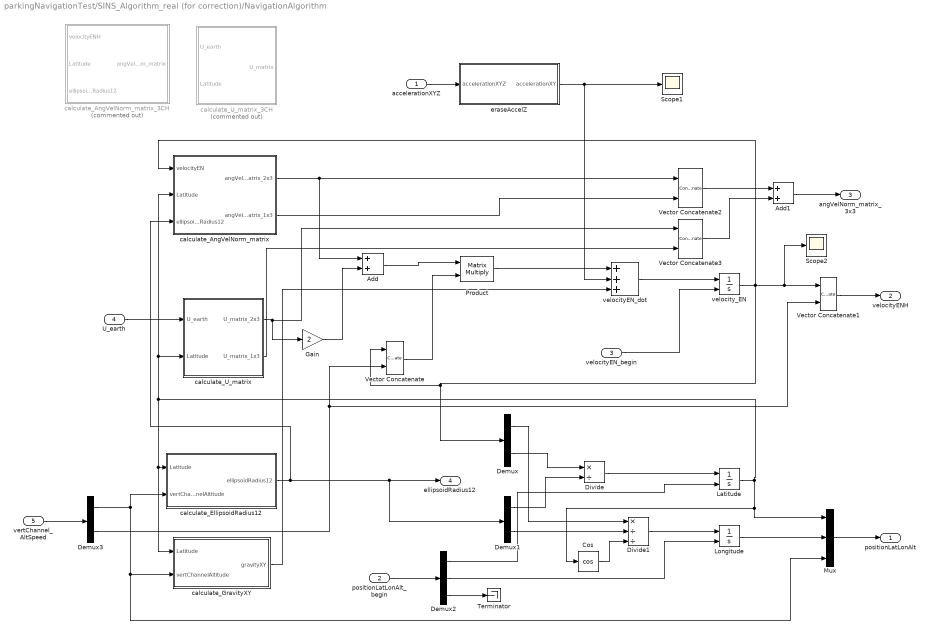
== system parkingNavigationTest/SINS_Algorithm_real (for correction)/NavigationAlgorithm ==
  accelerationXYZ : Inport
  positionLatLonAlt_begin : Inport  Port=2
  velocityEN_begin : Inport  Port=3
  U_earth : Inport  Port=4
  vertChannel_AltSpeed : Inport  Port=5
  Add : Sum
  Add1 : Sum
  Cos : Trigonometry  Operator=cos
  Demux : Demux  Outputs=2
  Demux1 : Demux  Outputs=2
  Demux2 : Demux  Outputs=3
  Demux3 : Demux  Outputs=2
  Divide : Product  Inputs=*/
  Divide1 : Product  Inputs=*//
  Gain : Gain  Gain=2
  Latitude : Integrator  InitialConditionSource=external
  Longitude : Integrator  InitialConditionSource=external
  Mux : Mux  Inputs=3
  Product : Product  Multiplication=Matrix(*)
  Scope1 : Scope
  Scope2 : Scope
  Terminator : Terminator
  Vector Concatenate{,1..3} (4 alike) : Concatenate  Mode=Multidimensional array
  calculate_AngVelNorm_matrix : Subsystem
  calculate_AngVelNorm_matrix_3CH : Subsystem  Commented=on
  calculate_EllipsoidRadius12 : Subsystem
  calculate_GravityXY : Subsystem
  calculate_U_matrix : Subsystem
  calculate_U_matrix_3CH : Subsystem  Commented=on
  eraseAccelZ : Subsystem
  velocityEN_dot : Sum  Inputs=+++
  velocity_EN : Integrator  InitialConditionSource=external  InitialCondition=[0; 0; 0]
  positionLatLonAlt : Outport
  velocityENH : Outport  Port=2
  angVelNorm_matrix_3x3 : Outport  Port=3
  ellipsoidRadius12 : Outport  Port=4
  wires:
  calculate_U_matrix/1(U_matrix_2x3) -> Vector Concatenate3/1, Gain/1
  calculate_AngVelNorm_matrix/1(angVelNorm_matrix_2x3) -> Vector Concatenate2/1, Add/1
  Gain/1 -> Add/2
  Add/1 -> Product/1
  Product/1 -> velocityEN_dot/1
  velocityEN_dot/1 -> velocity_EN/1
  Divide/1 -> Latitude/1
  Demux/2 -> Divide/1
  Demux1/1 -> Divide/2
  Latitude/1 -> calculate_GravityXY/1(Latitude), calculate_EllipsoidRadius12/1(Latitude), calculate_U_matrix/2(Latitude), calculate_AngVelNorm_matrix/2(Latitude), Mux/1, Cos/1
  Divide1/1 -> Longitude/1
  Demux/1 -> Divide1/1
  Demux1/2 -> Divide1/2
  Cos/1 -> Divide1/3
  Longitude/1 -> Mux/2
  Demux3/1 -> Mux/3, calculate_GravityXY/2(vertChannelAltitude), calculate_EllipsoidRadius12/2(vertChannelAltitude)
  calculate_EllipsoidRadius12/1(ellipsoidRadius12) -> calculate_AngVelNorm_matrix/3(ellipsoidRadius12), ellipsoidRadius12/1, Demux1/1
  U_earth/1 -> calculate_U_matrix/1(U_earth)
  Mux/1 -> positionLatLonAlt/1
  velocity_EN/1 -> Scope2/1, Vector Concatenate1/1, calculate_AngVelNorm_matrix/1(velocityEN), Vector Concatenate/1, Demux/1
  calculate_GravityXY/1(gravityXY) -> velocityEN_dot/3
  positionLatLonAlt_begin/1 -> Demux2/1
  Demux2/1 -> Latitude/2
  Demux2/2 -> Longitude/2
  velocityEN_begin/1 -> velocity_EN/2
  vertChannel_AltSpeed/1 -> Demux3/1
  Demux3/2 -> Vector Concatenate1/2, Vector Concatenate/2
  Vector Concatenate/1 -> Product/2
  Vector Concatenate1/1 -> velocityENH/1
  calculate_AngVelNorm_matrix/2(angVelNorm_matrix_1x3) -> Vector Concatenate2/2
  accelerationXYZ/1 -> eraseAccelZ/1(accelerationXYZ)
  eraseAccelZ/1(accelerationXY) -> Scope1/1, velocityEN_dot/2
  Demux2/3 -> Terminator/1
  calculate_U_matrix/2(U_matrix_1x3) -> Vector Concatenate3/2
  Vector Concatenate2/1 -> Add1/1
  Vector Concatenate3/1 -> Add1/2
  Add1/1 -> angVelNorm_matrix_3x3/1

== system parkingNavigationTest/SINS_Algorithm_real (for correction)/OrientationAlgorithm ==
  angVel_inertial_assoc : Inport
  angVelNorm_matrix : Inport  Port=2
  C_assoc_norm_begin : Inport  Port=3
  C to Orientation Angles : Subsystem
  Demux : Demux  Outputs=3
  Integrator : Integrator  InitialConditionSource=external  InitialCondition=[0, 0, 0; 0, 0, 0; 0, 0, 0]
  Product : Product  Multiplication=Matrix(*)
  Product1 : Product  Multiplication=Matrix(*)
  "Skew symmetric matrix " : Subsystem
  Sum : Sum  Inputs=+-
  Transpose : matrix_library/Transpose
      settings: SourceProductBaseCode=SL
  C_assoc_norm : Outport
  RollPitchYaw : Outport  Port=2
  wires:
  angVel_inertial_assoc/1 -> Demux/1
  angVelNorm_matrix/1 -> Transpose/1
  Sum/1 -> Integrator/1
  Transpose/1 -> Product1/1
  Product/1 -> Sum/1
  Product1/1 -> Sum/2
  Integrator/1 -> C to Orientation Angles/1(C), Product/1, Product1/2, C_assoc_norm/1
  C to Orientation Angles/1(RollPitchYaw) -> RollPitchYaw/1
  Demux/2 -> "Skew symmetric matrix "/2(angVel_y)
  Demux/1 -> "Skew symmetric matrix "/1(angVel_x)
  Demux/3 -> "Skew symmetric matrix "/3(angVel_z)
  "Skew symmetric matrix "/1(angVel_matrix) -> Product/2
  C_assoc_norm_begin/1 -> Integrator/2

== system parkingNavigationTest/SINS_Algorithm_real (for correction)/removeVelocityH ==
  velocityENH_begin : Inport
  Demux : Demux  Outputs=3
  Mux : Mux  Inputs=2
  Terminator : Terminator
  velocityEN_begin : Outport
  wires:
  velocityENH_begin/1 -> Demux/1
  Demux/1 -> Mux/1
  Demux/2 -> Mux/2
  Mux/1 -> velocityEN_begin/1
  Demux/3 -> Terminator/1

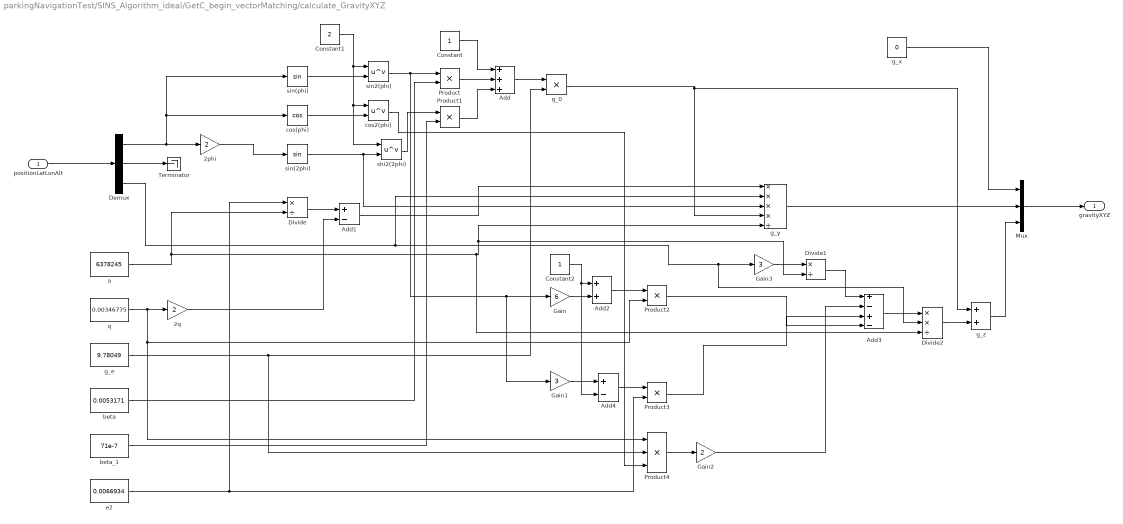
== system parkingNavigationTest/SINS_Algorithm_ideal/GetC_begin_vectorMatching/calculate_GravityXYZ ==
  positionLatLonAlt : Inport
  2phi : Gain  Gain=2
  2q : Gain  Gain=2
  Add : Sum  Inputs=+++
  Add1 : Sum  Inputs=+-
  Add2 : Sum
  Add3 : Sum  Inputs=+-+-
  Add4 : Sum  Inputs=+-
  Constant : Constant
  Constant1 : Constant  Value=2
  Constant2 : Constant
  Demux : Demux  Outputs=3
  Divide : Product  Inputs=*/
  Divide1 : Product  Inputs=*/
  Divide2 : Product  Inputs=**/
  Gain : Gain  Gain=6
  Gain1 : Gain  Gain=3
  Gain2 : Gain  Gain=2
  Gain3 : Gain  Gain=3
  Mux : Mux  Inputs=3
  Product{,1..3} (4 alike) : Product
  Product4 : Product  Inputs=3
  Terminator : Terminator
  a : Constant  Value=6378245
  beta : Constant  Value=0.0053171
  beta_1 : Constant  Value=71e-7
  cos(phi) : Trigonometry  Operator=cos
  cos2(phi) : Math  Operator=pow  SaturateOnIntegerOverflow=on
  e2 : Constant  Value=0.0066934
  g_0 : Product
  g_e : Constant  Value=9.78049
  g_x : Constant  Value=0
  g_y : Product  Inputs=****/
  g_z : Sum
  q : Constant  Value=0.00346775
  shi2(2phi) : Math  Operator=pow  SaturateOnIntegerOverflow=on
  sin(2phi) : Trigonometry
  sin(phi) : Trigonometry
  sin2(phi) : Math  Operator=pow  SaturateOnIntegerOverflow=on
  gravityXYZ : Outport
  wires:
  positionLatLonAlt/1 -> Demux/1
  Demux/2 -> Terminator/1
  Mux/1 -> gravityXYZ/1
  Demux/1 -> cos(phi)/1, sin(phi)/1, 2phi/1
  2phi/1 -> sin(2phi)/1
  sin(phi)/1 -> sin2(phi)/2
  Constant1/1 -> cos2(phi)/1, shi2(2phi)/1, sin2(phi)/1
  sin(2phi)/1 -> g_y/3, shi2(2phi)/2
  beta/1 -> Product/2
  sin2(phi)/1 -> Gain1/1, Gain/1, Product/1
  shi2(2phi)/1 -> Product1/1
  beta_1/1 -> Product1/2
  Product/1 -> Add/2
  Constant/1 -> Add/1
  Product1/1 -> Add/3
  Add/1 -> g_0/1
  g_e/1 -> Product4/2, g_0/2
  e2/1 -> Product3/2, Divide/1
  a/1 -> Divide2/3, Divide1/2, g_y/5, Divide/2
  Divide/1 -> Add1/1
  q/1 -> Product4/1, Product2/2, 2q/1
  2q/1 -> Add1/2
  Add1/1 -> g_y/1
  Demux/3 -> g_y/2, Divide2/2, Gain3/1
  g_0/1 -> g_z/1, g_y/4
  g_y/1 -> Mux/2
  cos(phi)/1 -> cos2(phi)/2
  Gain/1 -> Add2/2
  Constant2/1 -> Add4/2, Add2/1
  Add2/1 -> Product2/1
  Product2/1 -> Add3/4
  Gain1/1 -> Add4/1
  Add4/1 -> Product3/1
  Product3/1 -> Add3/3
  Product4/1 -> Gain2/1
  cos2(phi)/1 -> Product4/3
  Gain2/1 -> Add3/2
  Gain3/1 -> Divide1/1
  Divide1/1 -> Add3/1
  Add3/1 -> Divide2/1
  Divide2/1 -> g_z/2
  g_z/1 -> Mux/3
  g_x/1 -> Mux/1

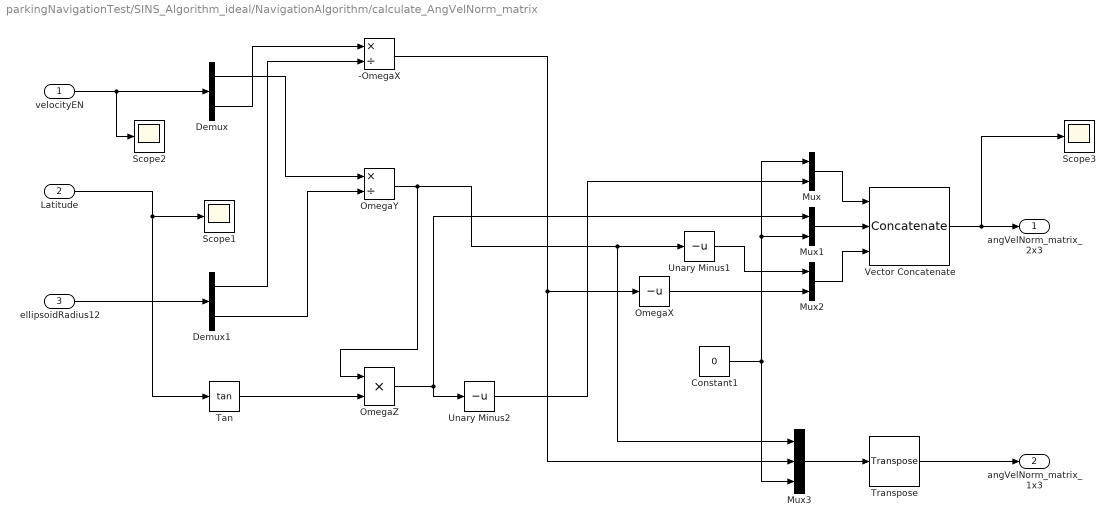
== system parkingNavigationTest/SINS_Algorithm_ideal/NavigationAlgorithm/calculate_AngVelNorm_matrix ==
  velocityEN : Inport
  Latitude : Inport  Port=2
  ellipsoidRadius12 : Inport  Port=3
  -OmegaX : Product  Inputs=*/
  Constant1 : Constant  Value=0
  Demux : Demux  Outputs=2
  Demux1 : Demux  Outputs=2
  Mux : Mux  Inputs=2
  Mux1 : Mux  Inputs=2
  Mux2 : Mux  Inputs=2
  Mux3 : Mux  Inputs=3
  OmegaX : UnaryMinus
  OmegaY : Product  Inputs=*/
  OmegaZ : Product  Inputs=**
  Scope1 : Scope
  Scope2 : Scope
  Scope3 : Scope
  Tan : Trigonometry  Operator=tan
  Transpose : matrix_library/Transpose
      settings: SourceProductBaseCode=SL
  Unary Minus1 : UnaryMinus
  Unary Minus2 : UnaryMinus
  Vector Concatenate : Concatenate  NumInputs=3  Mode=Multidimensional array  ConcatenateDimension=2
  angVelNorm_matrix_2x3 : Outport
  angVelNorm_matrix_1x3 : Outport  Port=2
  wires:
  velocityEN/1 -> Scope2/1, Demux/1
  ellipsoidRadius12/1 -> Demux1/1
  Demux/2 -> -OmegaX/1
  Demux1/1 -> -OmegaX/2
  -OmegaX/1 -> Mux3/2, OmegaX/1
  OmegaX/1 -> Mux2/2
  Demux/1 -> OmegaY/1
  Demux1/2 -> OmegaY/2
  OmegaY/1 -> OmegaZ/1, Mux3/1, Unary Minus1/1
  Unary Minus1/1 -> Mux2/1
  Tan/1 -> OmegaZ/2
  Latitude/1 -> Scope1/1, Tan/1
  OmegaZ/1 -> Unary Minus2/1, Mux1/1
  Unary Minus2/1 -> Mux/2
  Constant1/1 -> Mux3/3, Mux/1, Mux1/2
  Mux1/1 -> Vector Concatenate/2
  Mux/1 -> Vector Concatenate/1
  Mux2/1 -> Vector Concatenate/3
  Vector Concatenate/1 -> Scope3/1, angVelNorm_matrix_2x3/1
  Mux3/1 -> Transpose/1
  Transpose/1 -> angVelNorm_matrix_1x3/1

== system parkingNavigationTest/SINS_Algorithm_ideal/NavigationAlgorithm/calculate_AngVelNorm_matrix_3CH ==
  velocityENH : Inport
  Latitude : Inport  Port=2
  ellipsoidRadius12 : Inport  Port=3
  Constant : Constant  Value=0
  Create 3x3 Matrix : sharedutil/Create 3x3 Matrix  aMode=aMode
      settings: SourceProductBaseCode=AE,PW,DR,MT,UV,VE
  Demux : Demux  Outputs=3
  Demux1 : Demux  Outputs=2
  Divide : Product  Inputs=*/
  OmegaX : UnaryMinus
  OmegaY : Product  Inputs=*/
  OmegaZ : Product  Inputs=**/
  Tan : Trigonometry  Operator=tan
  Terminator : Terminator
  Unary Minus1 : UnaryMinus
  Unary Minus2 : UnaryMinus
  angVelNorm_matrix : Outport
  wires:
  velocityENH/1 -> Demux/1
  ellipsoidRadius12/1 -> Demux1/1
  Demux/2 -> Divide/1
  Demux1/1 -> Divide/2
  Divide/1 -> Create 3x3 Matrix/8, OmegaX/1
  OmegaX/1 -> Create 3x3 Matrix/6
  Demux/1 -> OmegaZ/1, OmegaY/1
  Demux1/2 -> OmegaZ/3, OmegaY/2
  OmegaY/1 -> Unary Minus1/1, Create 3x3 Matrix/7
  Unary Minus1/1 -> Create 3x3 Matrix/3
  Tan/1 -> OmegaZ/2
  Latitude/1 -> Tan/1
  OmegaZ/1 -> Unary Minus2/1, Create 3x3 Matrix/2
  Unary Minus2/1 -> Create 3x3 Matrix/4
  Constant/1 -> Create 3x3 Matrix/9, Create 3x3 Matrix/5, Create 3x3 Matrix/1
  Create 3x3 Matrix/1 -> angVelNorm_matrix/1
  Demux/3 -> Terminator/1

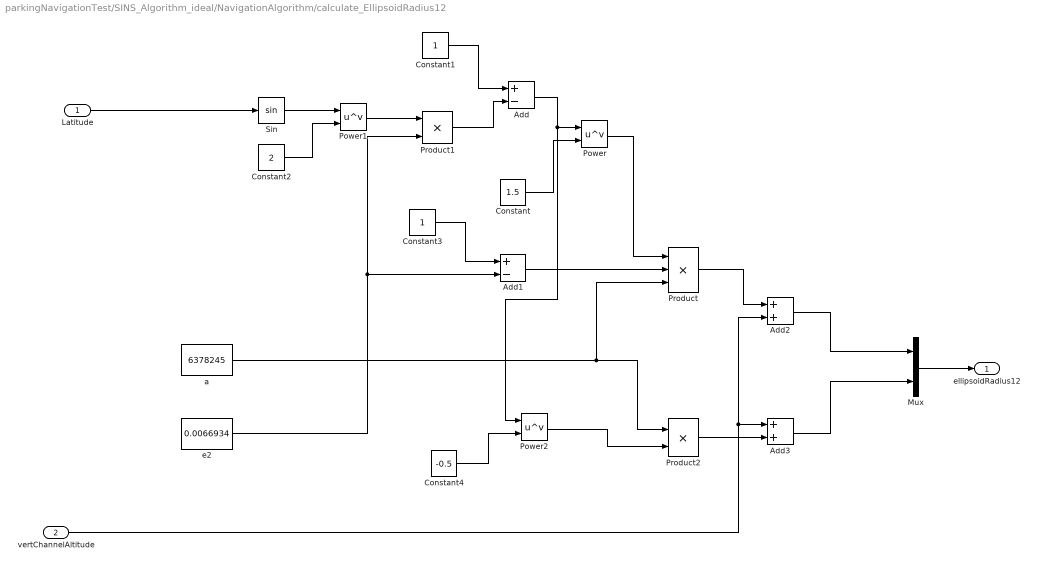
== system parkingNavigationTest/SINS_Algorithm_ideal/NavigationAlgorithm/calculate_EllipsoidRadius12 ==
  Latitude : Inport
  vertChannelAltitude : Inport  Port=2
  Add : Sum  Inputs=+-
  Add1 : Sum  Inputs=+-
  Add2 : Sum
  Add3 : Sum
  Constant : Constant  Value=1.5
  Constant1 : Constant
  Constant2 : Constant  Value=2
  Constant3 : Constant
  Constant4 : Constant  Value=-0.5
  Mux : Mux  Inputs=2
  Power : Math  Operator=pow  SaturateOnIntegerOverflow=on
  Power1 : Math  Operator=pow  SaturateOnIntegerOverflow=on
  Power2 : Math  Operator=pow  SaturateOnIntegerOverflow=on
  Product : Product  Inputs=3
  Product1 : Product
  Product2 : Product
  Sin : Trigonometry
  a : Constant  Value=6378245
  e2 : Constant  Value=0.0066934
  ellipsoidRadius12 : Outport
  wires:
  Mux/1 -> ellipsoidRadius12/1
  Constant1/1 -> Add/1
  Product1/1 -> Add/2
  Power1/1 -> Product1/1
  Sin/1 -> Power1/1
  Constant2/1 -> Power1/2
  Latitude/1 -> Sin/1
  e2/1 -> Add1/2, Product1/2
  Add/1 -> Power2/1, Power/1
  Constant/1 -> Power/2
  Power/1 -> Product/1
  Constant3/1 -> Add1/1
  Add1/1 -> Product/2
  a/1 -> Product2/1, Product/3
  Product/1 -> Add2/1
  vertChannelAltitude/1 -> Add2/2, Add3/1
  Add2/1 -> Mux/1
  Constant4/1 -> Power2/2
  Power2/1 -> Product2/2
  Product2/1 -> Add3/2
  Add3/1 -> Mux/2

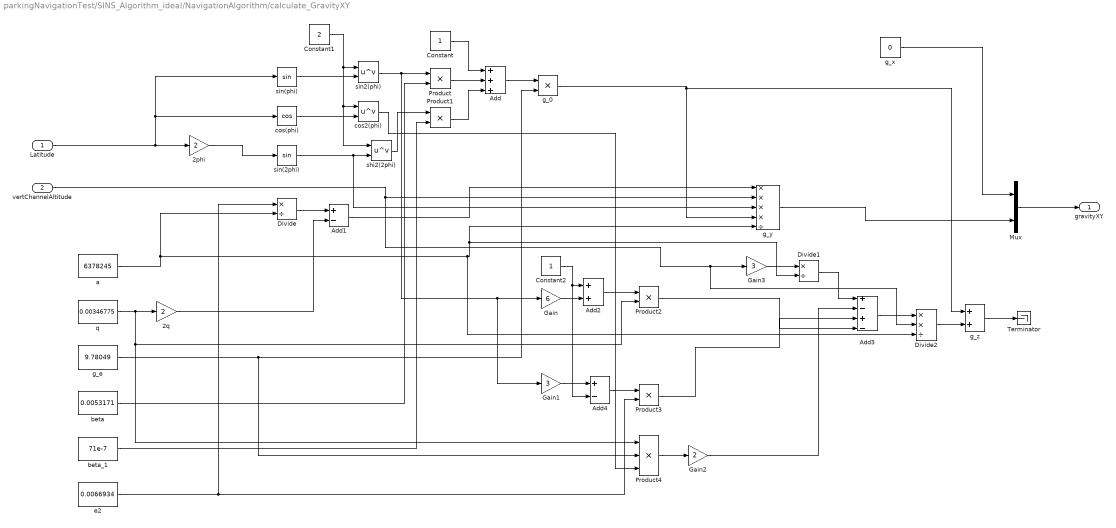
== system parkingNavigationTest/SINS_Algorithm_ideal/NavigationAlgorithm/calculate_GravityXY ==
  Latitude : Inport
  vertChannelAltitude : Inport  Port=2
  2phi : Gain  Gain=2
  2q : Gain  Gain=2
  Add : Sum  Inputs=+++
  Add1 : Sum  Inputs=+-
  Add2 : Sum
  Add3 : Sum  Inputs=+-+-
  Add4 : Sum  Inputs=+-
  Constant : Constant
  Constant1 : Constant  Value=2
  Constant2 : Constant
  Divide : Product  Inputs=*/
  Divide1 : Product  Inputs=*/
  Divide2 : Product  Inputs=**/
  Gain : Gain  Gain=6
  Gain1 : Gain  Gain=3
  Gain2 : Gain  Gain=2
  Gain3 : Gain  Gain=3
  Mux : Mux  Inputs=2
  Product{,1..3} (4 alike) : Product
  Product4 : Product  Inputs=3
  Terminator : Terminator
  a : Constant  Value=6378245
  beta : Constant  Value=0.0053171
  beta_1 : Constant  Value=71e-7
  cos(phi) : Trigonometry  Operator=cos
  cos2(phi) : Math  Operator=pow  SaturateOnIntegerOverflow=on
  e2 : Constant  Value=0.0066934
  g_0 : Product
  g_e : Constant  Value=9.78049
  g_x : Constant  Value=0
  g_y : Product  Inputs=****/
  g_z : Sum
  q : Constant  Value=0.00346775
  shi2(2phi) : Math  Operator=pow  SaturateOnIntegerOverflow=on
  sin(2phi) : Trigonometry
  sin(phi) : Trigonometry
  sin2(phi) : Math  Operator=pow  SaturateOnIntegerOverflow=on
  gravityXY : Outport
  wires:
  Mux/1 -> gravityXY/1
  Latitude/1 -> cos(phi)/1, sin(phi)/1, 2phi/1
  2phi/1 -> sin(2phi)/1
  sin(phi)/1 -> sin2(phi)/2
  Constant1/1 -> cos2(phi)/1, shi2(2phi)/1, sin2(phi)/1
  sin(2phi)/1 -> g_y/3, shi2(2phi)/2
  beta/1 -> Product/2
  sin2(phi)/1 -> Gain1/1, Gain/1, Product/1
  shi2(2phi)/1 -> Product1/1
  beta_1/1 -> Product1/2
  Product/1 -> Add/2
  Constant/1 -> Add/1
  Product1/1 -> Add/3
  Add/1 -> g_0/1
  g_e/1 -> Product4/2, g_0/2
  e2/1 -> Product3/2, Divide/1
  a/1 -> Divide2/3, Divide1/2, g_y/5, Divide/2
  Divide/1 -> Add1/1
  q/1 -> Product4/1, Product2/2, 2q/1
  2q/1 -> Add1/2
  Add1/1 -> g_y/1
  vertChannelAltitude/1 -> Divide2/2, Gain3/1, g_y/2
  g_0/1 -> g_z/1, g_y/4
  g_y/1 -> Mux/2
  cos(phi)/1 -> cos2(phi)/2
  Gain/1 -> Add2/2
  Constant2/1 -> Add4/2, Add2/1
  Add2/1 -> Product2/1
  Product2/1 -> Add3/4
  Gain1/1 -> Add4/1
  Add4/1 -> Product3/1
  Product3/1 -> Add3/3
  Product4/1 -> Gain2/1
  cos2(phi)/1 -> Product4/3
  Gain2/1 -> Add3/2
  Gain3/1 -> Divide1/1
  Divide1/1 -> Add3/1
  Add3/1 -> Divide2/1
  Divide2/1 -> g_z/2
  g_z/1 -> Terminator/1
  g_x/1 -> Mux/1

== system parkingNavigationTest/SINS_Algorithm_ideal/NavigationAlgorithm/calculate_U_matrix ==
  U_earth : Inport
  Latitude : Inport  Port=2
  Constant : Constant  Value=0
  Cos : Trigonometry  Operator=cos
  Mux : Mux  Inputs=2
  Mux1 : Mux  Inputs=2
  Mux2 : Mux  Inputs=2
  Mux3 : Mux  Inputs=3
  Sin : Trigonometry
  Transpose : matrix_library/Transpose
      settings: SourceProductBaseCode=SL
  U_y : Product
  U_z : Product
  Unary Minus : UnaryMinus
  Unary Minus1 : UnaryMinus
  Vector Concatenate : Concatenate  NumInputs=3  Mode=Multidimensional array  ConcatenateDimension=2
  U_matrix_2x3 : Outport
  U_matrix_1x3 : Outport  Port=2
  wires:
  Latitude/1 -> Sin/1, Cos/1
  U_earth/1 -> U_z/1, U_y/1
  Cos/1 -> U_y/2
  U_y/1 -> Mux3/1, Unary Minus/1
  Unary Minus/1 -> Mux2/1
  Sin/1 -> U_z/2
  U_z/1 -> Mux1/1, Unary Minus1/1
  Unary Minus1/1 -> Mux/2
  Mux/1 -> Vector Concatenate/1
  Mux2/1 -> Vector Concatenate/3
  Mux1/1 -> Vector Concatenate/2
  Constant/1 -> Mux3/3, Mux3/2, Mux/1, Mux1/2, Mux2/2
  Vector Concatenate/1 -> U_matrix_2x3/1
  Mux3/1 -> Transpose/1
  Transpose/1 -> U_matrix_1x3/1

== system parkingNavigationTest/SINS_Algorithm_ideal/NavigationAlgorithm/calculate_U_matrix_3CH ==
  U_earth : Inport
  Latitude : Inport  Port=2
  Constant : Constant  Value=0
  Cos : Trigonometry  Operator=cos
  Create 3x3 Matrix : sharedutil/Create 3x3 Matrix  aMode=aMode
      settings: SourceProductBaseCode=AE,PW,DR,MT,UV,VE
  Product : Product
  Product1 : Product
  Sin : Trigonometry
  Unary Minus : UnaryMinus
  Unary Minus1 : UnaryMinus
  U_matrix : Outport
  wires:
  Latitude/1 -> Sin/1, Cos/1
  U_earth/1 -> Product1/1, Product/1
  Cos/1 -> Product/2
  Product/1 -> Unary Minus/1, Create 3x3 Matrix/7
  Unary Minus/1 -> Create 3x3 Matrix/3
  Sin/1 -> Product1/2
  Product1/1 -> Unary Minus1/1, Create 3x3 Matrix/2
  Unary Minus1/1 -> Create 3x3 Matrix/4
  Constant/1 -> Create 3x3 Matrix/9, Create 3x3 Matrix/8, Create 3x3 Matrix/6, Create 3x3 Matrix/5, Create 3x3 Matrix/1
  Create 3x3 Matrix/1 -> U_matrix/1

== system parkingNavigationTest/SINS_Algorithm_ideal/NavigationAlgorithm/eraseAccelZ ==
  accelerationXYZ : Inport
  Demux : Demux  Outputs=3
  Mux : Mux  Inputs=2
  Terminator : Terminator
  accelerationXY : Outport
  wires:
  accelerationXYZ/1 -> Demux/1
  Demux/1 -> Mux/1
  Demux/2 -> Mux/2
  Mux/1 -> accelerationXY/1
  Demux/3 -> Terminator/1

== system parkingNavigationTest/SINS_Algorithm_ideal/OrientationAlgorithm/C to Orientation Angles ==
  C : Inport
  "C(1, 1)" : Selector  NumberOfDimensions=2  InputPortWidth=3  IndexOptions=Index vector (dialog),Index vector (dialog)  Indices=1,1  OutputSizes=1,1
  "C(2, 1)" : Selector  NumberOfDimensions=2  InputPortWidth=3  IndexOptions=Index vector (dialog),Index vector (dialog)  Indices=2,1  OutputSizes=1,1
  "C(2, 2)" : Selector  NumberOfDimensions=2  InputPortWidth=3  IndexOptions=Index vector (dialog),Index vector (dialog)  Indices=2,2  OutputSizes=1,1
  "C(2, 3)" : Selector  NumberOfDimensions=2  InputPortWidth=3  IndexOptions=Index vector (dialog),Index vector (dialog)  Indices=2,3  OutputSizes=1,1
  "C(3, 1)" : Selector  NumberOfDimensions=2  InputPortWidth=3  IndexOptions=Index vector (dialog),Index vector (dialog)  Indices=3,1  OutputSizes=1,1
  Divide2 : Product  Inputs=*/
  Divide3 : Product  Inputs=*/
  Mux : Mux  Inputs=3
  Sin3 : Trigonometry  Operator=atan
  Sin4 : Trigonometry  Operator=atan
  Sin5 : Trigonometry  Operator=asin
  Unary Minus : UnaryMinus
  Unary Minus3 : UnaryMinus
  RollPitchYaw : Outport
  wires:
  Divide2/1 -> Sin3/1
  "C(2, 2)"/1 -> Divide2/2
  Divide3/1 -> Sin4/1
  "C(3, 1)"/1 -> Unary Minus3/1
  Sin3/1 -> Mux/1
  Mux/1 -> RollPitchYaw/1
  C/1 -> "C(2, 3)"/1, "C(2, 2)"/1, "C(2, 1)"/1, "C(3, 1)"/1, "C(1, 1)"/1
  "C(1, 1)"/1 -> Divide3/2
  "C(2, 1)"/1 -> Sin5/1
  Unary Minus3/1 -> Divide3/1
  "C(2, 3)"/1 -> Unary Minus/1
  Unary Minus/1 -> Divide2/1
  Sin5/1 -> Mux/2
  Sin4/1 -> Mux/3

== system parkingNavigationTest/SINS_Algorithm_ideal/OrientationAlgorithm/Skew symmetric matrix  ==
  angVel_x : Inport
  angVel_y : Inport  Port=2
  angVel_z : Inport  Port=3
  Constant5 : Constant  Value=0
  Mux1 : Mux  Inputs=3
  Mux2 : Mux  Inputs=3
  Mux3 : Mux  Inputs=3
  Unary Minus1 : UnaryMinus
  Unary Minus2 : UnaryMinus
  Unary Minus6 : UnaryMinus
  get angVel_matrix : Concatenate  NumInputs=3  Mode=Multidimensional array  ConcatenateDimension=2
  angVel_matrix : Outport
  wires:
  Mux3/1 -> get angVel_matrix/3
  Unary Minus1/1 -> Mux3/2
  Unary Minus2/1 -> Mux1/3
  angVel_x/1 -> Mux2/3, Unary Minus1/1
  get angVel_matrix/1 -> angVel_matrix/1
  Constant5/1 -> Mux3/3, Mux2/2, Mux1/1
  Mux1/1 -> get angVel_matrix/1
  Mux2/1 -> get angVel_matrix/2
  angVel_y/1 -> Unary Minus2/1, Mux3/1
  Unary Minus6/1 -> Mux2/1
  angVel_z/1 -> Unary Minus6/1, Mux1/2
